simulink model "Aero_Var120"  (R2016b)
settings: Solver=VariableStepAuto  StartTime=0.0  StopTime=10.0  RelTol=1e-3
undefined symbols (not defined in the file or in its folder): AC
libraries: OpenFlightUtilLib x3, simulink x1
settings Model: Creator=UAVLAB  LastModifiedBy=rega0051
settings DataIOCC: ExternalInput=simIn  InitialState=simStateInit  SaveOutput=off  SignalLogging=off  DSMLogging=off  SaveTime=off  StateSaveName=simStates  TimeSaveName=simTime  OutputSaveName=simOut  SignalLoggingName=simLog  DSMLoggingName=simData

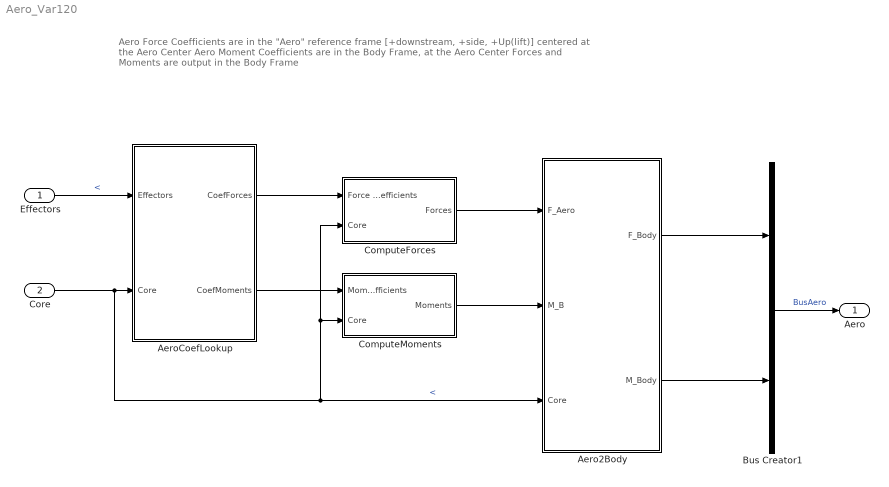
== system Aero_Var120 ==
  note: Aero Force Coefficients are in the "Aero" reference frame [+downstream, +side, +Up(lift)] centered at the Aero Center
      | Aero Moment Coefficients are in the Body Frame, at the Aero Center
      |
      | Forces and Moments are output in the Body Frame
  Effectors : Inport  OutDataTypeStr=Bus: BusEff
      settings: AttributesFormatString=%<OutDataTypeStr>
  Core : Inport  Port=2  OutDataTypeStr=Bus: BusCore
      settings: AttributesFormatString=%<OutDataTypeStr>
  Aero2Body : Subsystem
  AeroCoefLookup : Subsystem
  Bus Creator1 : BusCreator  Inputs=2  OutDataTypeStr=Bus: BusAero
      settings: AttributesFormatString=%<OutDataTypeStr>
  ComputeForces : Subsystem
  ComputeMoments : Subsystem
  Aero : Outport  OutDataTypeStr=Bus: BusAero
      settings: AttributesFormatString=%<OutDataTypeStr>
  wires:
  Effectors/1 -> AeroCoefLookup/1(Effectors)  "<"
  ComputeForces/1(Forces) -> Aero2Body/1(F_Aero)
  ComputeMoments/1(Moments) -> Aero2Body/2(M_B)
  Aero2Body/1(F_Body) -> Bus Creator1/1
  Aero2Body/2(M_Body) -> Bus Creator1/2
  AeroCoefLookup/1(CoefForces) -> ComputeForces/1(Force Coefficients)
  AeroCoefLookup/2(CoefMoments) -> ComputeMoments/1(Moment Coefficients)
  Bus Creator1/1 -> Aero/1  "BusAero"
  Core/1 -> AeroCoefLookup/2(Core), ComputeForces/2(Core), ComputeMoments/2(Core), Aero2Body/3(Core)  "<"

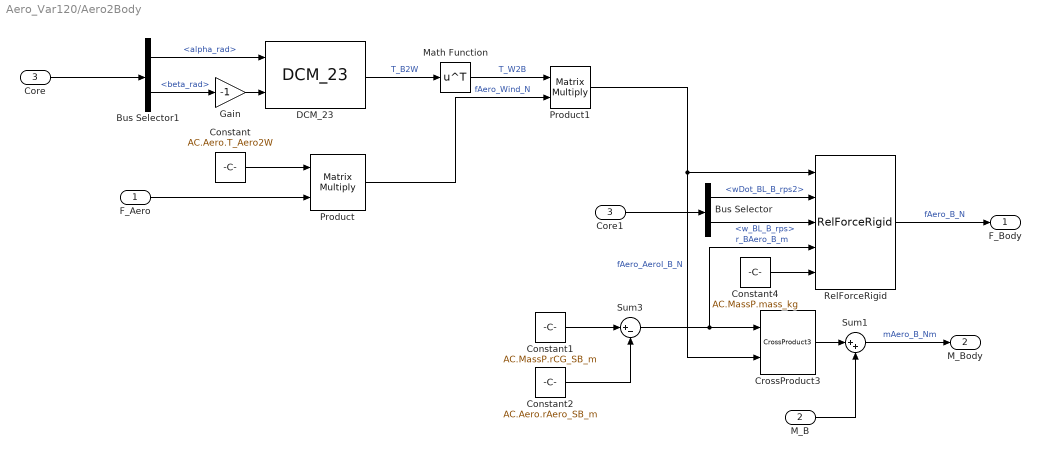
== system Aero_Var120/Aero2Body ==
  F_Aero : Inport
  M_B : Inport  Port=2
  Core : Inport  Port=3
  Bus Selector : BusSelector  OutputSignals=BusEom.wDot_BL_B_rps2,BusEom.w_BL_B_rps
  Bus Selector1 : BusSelector  OutputSignals=BusAux.BusFlow.alpha_rad,BusAux.BusFlow.beta_rad
  Constant : Constant  Value=AC.Aero.T_Aero2W
      settings: AttributesFormatString=%<Value>
  Constant1 : Constant  Value=AC.MassP.rCG_SB_m
      settings: AttributesFormatString=%<Value>
  Constant2 : Constant  Value=AC.Aero.rAero_SB_m
      settings: AttributesFormatString=%<Value>
  Constant4 : Constant  Value=AC.MassP.mass_kg
      settings: AttributesFormatString=%<Value>
  Core1 : InportShadow  Port=3
  CrossProduct3 : OpenFlightUtilLib/Math/CrossProduct3
  DCM_23 : OpenFlightUtilLib/Transformations/DCM_23
  Gain : Gain  Gain=-1
  Math Function : Math  Operator=transpose  SaturateOnIntegerOverflow=on
  Product : Product  Multiplication=Matrix(*)  RndMeth=Zero
  Product1 : Product  Multiplication=Matrix(*)  RndMeth=Zero
  RelForceRigid : OpenFlightUtilLib/Kinematics and Dynamics/RelForceRigid
  Sum1 : Sum  Inputs=|++  SaturateOnIntegerOverflow=on
  Sum3 : Sum  Inputs=|+-  SaturateOnIntegerOverflow=on
  F_Body : Outport
  M_Body : Outport  Port=2
  wires:
  Constant1/1 -> Sum3/1
  Constant2/1 -> Sum3/2
  Bus Selector/1 -> RelForceRigid/2  "<wDot_BL_B_rps2>"
  Bus Selector/2 -> RelForceRigid/3  "<w_BL_B_rps>"
  F_Aero/1 -> Product/2
  Constant/1 -> Product/1
  Core/1 -> Bus Selector1/1
  Math Function/1 -> Product1/1  "T_W2B"
  DCM_23/1 -> Math Function/1  "T_B2W"
  Product/1 -> Product1/2  "fAero_Wind_N"
  Product1/1 -> CrossProduct3/2, RelForceRigid/1  "fAero_AeroI_B_N"
  Sum3/1 -> RelForceRigid/4, CrossProduct3/1  "r_BAero_B_m"
  Core1/1 -> Bus Selector/1
  RelForceRigid/1 -> F_Body/1  "fAero_B_N"
  M_B/1 -> Sum1/2
  CrossProduct3/1 -> Sum1/1
  Sum1/1 -> M_Body/1  "mAero_B_Nm"
  Constant4/1 -> RelForceRigid/5
  Bus Selector1/1 -> DCM_23/1  "<alpha_rad>"
  Bus Selector1/2 -> Gain/1  "<beta_rad>"
  Gain/1 -> DCM_23/2

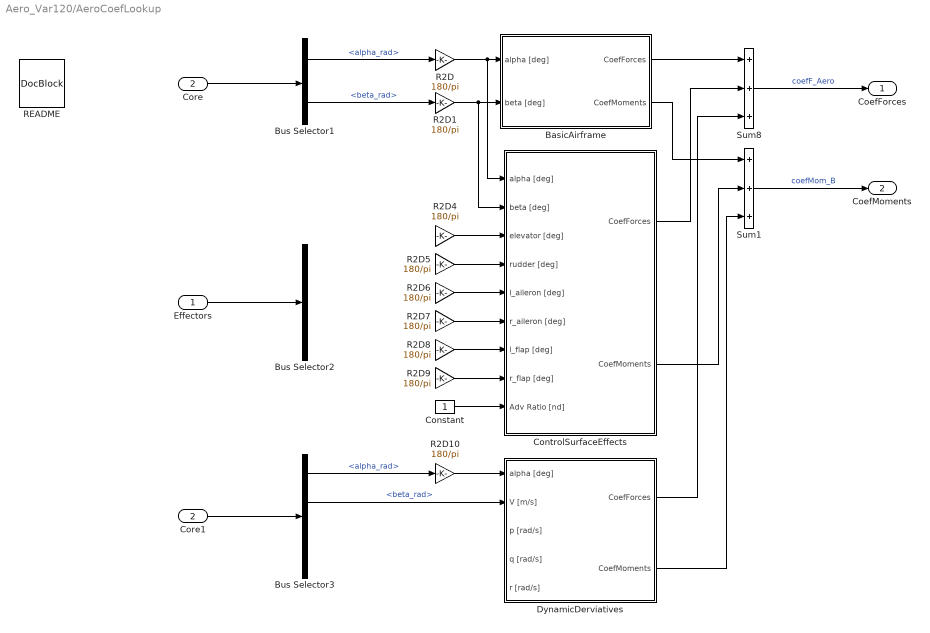
== system Aero_Var120/AeroCoefLookup ==
  Effectors : Inport
  Core : Inport  Port=2
  BasicAirframe : Subsystem
  Bus Selector1 : BusSelector  OutputSignals=BusAux.BusFlow.alpha_rad,BusAux.BusFlow.beta_rad
  Bus Selector2 : BusSelector  OutputSignals=BusSurf
  Bus Selector3 : BusSelector  OutputSignals=BusAux.BusFlow.alpha_rad,BusAux.BusFlow.beta_rad,BusAux.BusFlow.alphaDot_rps,BusAux.BusFlow.betaDot_rps
  Constant : Constant
  ControlSurfaceEffects : Subsystem
  Core1 : InportShadow  Port=2
  DynamicDerviatives : Subsystem
  R2D{,1,4..10} (9 alike) : Gain  Gain=180/pi
  README : simulink/Model-Wide Utilities/DocBlock  DocumentType=Text
      content=|
      | FASER Aerodynamic Model
      |
      | This block models the FASER aerodynamics using a nonlinear, lookup table
      | based, incremental aerodynamic model. This model is based on wind tunnel
      | data obtained from NASA Langley Research Center's 12-Foot Low Speed
      | Tunnel in 2006 and 2011. In general, the baseline aerodynamics are
      | modeled as a nonlinear function of angle of attack and sideslip angle.
      | Control surface effects are modeled as nonlinear functions of angle of
      | attack, sideslip angle, control surface deflection, and advance ratio.
      | Thrust effects are also modeled. DATCOM estimates of linear dynamic
      | derivatives are used for the pitch damping (Cmq), while the effect of
      | roll and yaw rate on CY, Cl, and Cn are modeled as nonlinear functions of
      | angle of attack and nondimensional rate based on forced oscilation wind
      | tunnel data.
      |
      | The effects of control surfaces and rates are modeled for only those
      | coefficients where there was a significant effect observed in the wind
      | tunnel data. They are listed here:
      |
      | Elevator: CD,CL,Cm
      | Rudder: CY,Cn
      | Aileron: Cl
      | Flaps: CD,CL,Cm
      | Thrust: All
      | Roll Rate (p): CY,Cl,Cn
      | Pitch Rate (q): Cm
      | Yaw Rate (r): CY,Cl,Cn
      |
      | The aero tables are stored in \Libraries\FASER_Aero.mat, and are loaded
      | into the aircraft configuration data structure (AC) when the FASER option
      | is input to UAV_config.m.
      |
      | >> AC.Aero
      |
      | ans =
      |
      |            dampder: [1x1 struct]
      |             C6_bas: [1x1 struct]
      |            dC1_ail: [1x1 struct]
      |            dC6_pow: [1x1 struct]
      |           dC3_flap: [1x1 struct]
      |            dC2_rud: [1x1 struct]
      |            dC3_ele: [1x1 struct]
      |              dC3_p: [1x1 struct]
      |              dC3_r: [1x1 struct]
      |     use_FASER_aero: 1
      |
      | The aero data is in the stability axis, so the six aero coefficients are
      | CL, CD, CY, Cl, Cm, Cn. The aero model uses a incremental approach; the
      | basic airframe is modeled in C6_bas; incremental (deltas) effects of
      | control surfaces, angular rate (dampder), and thrust are then added. The
      | form of the data structures is generally as follows:
      |
      | >> AC.Aero.C6_bas
      |
      | ans =
      |
      |      data: [16x13x6 double]
      |     alpha: [-5 0 5 10 11.7500 12.5000 13.2500 13.5000 15 16 17.5000 20 25 30 35 40]
      |      beta: [-30 -25 -20 -15 -10 -5 0 5 10 15 20 25 30]
      |       dim: 'Dimensions are [alpha]x[beta]x[CD,CY,CL,Cl,Cm,Cn]'
      |
      | Currently, the thrust effects are disabled (by setting the advance ratio
      | input to 1), as the current motor model does not output advance ratio.
      |
      | Note on table implementation: pre-lookups on the table indices (eg alpha,
      | beta, etc) are done to increase the speed of the simulation.
  Sum1 : Sum  Inputs=+++  SaturateOnIntegerOverflow=on  InputSameDT=on  OutDataTypeStr=Inherit: Same as first input
  Sum8 : Sum  Inputs=+++  SaturateOnIntegerOverflow=on  InputSameDT=on  OutDataTypeStr=Inherit: Same as first input
  CoefForces : Outport
  CoefMoments : Outport  Port=2
  wires:
  Sum1/1 -> CoefMoments/1  "coefMom_B"
  Sum8/1 -> CoefForces/1  "coefF_Aero"
  Effectors/1 -> Bus Selector2/1
  R2D10/1 -> DynamicDerviatives/1(alpha [deg])
  ? -> DynamicDerviatives/5(r [rad/s])
  ? -> DynamicDerviatives/4(q [rad/s])
  ? -> DynamicDerviatives/3(p [rad/s])
  ? -> R2D4/1
  Constant/1 -> ControlSurfaceEffects/9(Adv Ratio [nd])
  R2D/1 -> ControlSurfaceEffects/1(alpha [deg]), BasicAirframe/1(alpha [deg])
  R2D1/1 -> ControlSurfaceEffects/2(beta [deg]), BasicAirframe/2(beta [deg])
  R2D4/1 -> ControlSurfaceEffects/3(elevator [deg])
  ? -> R2D5/1
  R2D5/1 -> ControlSurfaceEffects/4(rudder [deg])
  ? -> R2D6/1
  ? -> R2D7/1
  ? -> R2D8/1
  ? -> R2D9/1
  R2D6/1 -> ControlSurfaceEffects/5(l_aileron [deg])
  R2D7/1 -> ControlSurfaceEffects/6(r_aileron [deg])
  R2D8/1 -> ControlSurfaceEffects/7(l_flap [deg])
  R2D9/1 -> ControlSurfaceEffects/8(r_flap [deg])
  Bus Selector1/2 -> R2D1/1  "<beta_rad>"
  Bus Selector1/1 -> R2D/1  "<alpha_rad>"
  Bus Selector3/1 -> R2D10/1  "<alpha_rad>"
  Bus Selector3/2 -> DynamicDerviatives/2(V [m/s])  "<beta_rad>"
  Core/1 -> Bus Selector1/1
  Core1/1 -> Bus Selector3/1
  BasicAirframe/1(CoefForces) -> Sum8/1
  ControlSurfaceEffects/1(CoefForces) -> Sum8/2
  DynamicDerviatives/1(CoefForces) -> Sum8/3
  BasicAirframe/2(CoefMoments) -> Sum1/1
  ControlSurfaceEffects/2(CoefMoments) -> Sum1/2
  DynamicDerviatives/2(CoefMoments) -> Sum1/3

== system Aero_Var120/ComputeForces ==
  Force Coefficients : Inport
  Core : Inport  Port=2
  Bus Selector : BusSelector  OutputSignals=BusAux.BusFlow.qBar_Pa
  Demux3 : Demux  Outputs=3
  Gain2 : Gain  Gain=AC.Aero.S  SaturateOnIntegerOverflow=on  OutDataTypeStr=Inherit: Same as input  ParamDataTypeStr=Inherit: Same as input
      settings: AttributesFormatString=%<Gain>
  Mux1 : Mux  Inputs=3
  Product6 : Product  SaturateOnIntegerOverflow=on  InputSameDT=on  OutDataTypeStr=Inherit: Same as first input
  Product7 : Product  SaturateOnIntegerOverflow=on  InputSameDT=on  OutDataTypeStr=Inherit: Same as first input
  Product8 : Product  SaturateOnIntegerOverflow=on  InputSameDT=on  OutDataTypeStr=Inherit: Same as first input
  Forces : Outport
  wires:
  Product6/1 -> Mux1/1  "fD_N"
  Product8/1 -> Mux1/3  "fL_N"
  Product7/1 -> Mux1/2  "fY_N"
  Mux1/1 -> Forces/1  "fAero_N"
  Demux3/2 -> Product7/1  "cY"
  Demux3/1 -> Product6/1  "cD"
  Demux3/3 -> Product8/1  "cL"
  Force Coefficients/1 -> Demux3/1
  Gain2/1 -> Product6/2, Product7/2, Product8/2
  Bus Selector/1 -> Gain2/1  "<qBar_Pa>"
  Core/1 -> Bus Selector/1

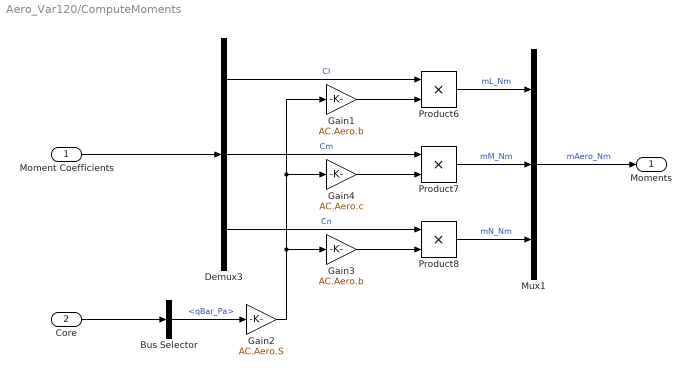
== system Aero_Var120/ComputeMoments ==
  Moment Coefficients : Inport
  Core : Inport  Port=2
  Bus Selector : BusSelector  OutputSignals=BusAux.BusFlow.qBar_Pa
  Demux3 : Demux  Outputs=3
  Gain1 : Gain  Gain=AC.Aero.b  SaturateOnIntegerOverflow=on  OutDataTypeStr=Inherit: Same as input  ParamDataTypeStr=Inherit: Same as input
      settings: AttributesFormatString=%<Gain>
  Gain2 : Gain  Gain=AC.Aero.S  SaturateOnIntegerOverflow=on  OutDataTypeStr=Inherit: Same as input  ParamDataTypeStr=Inherit: Same as input
      settings: AttributesFormatString=%<Gain>
  Gain3 : Gain  Gain=AC.Aero.b  SaturateOnIntegerOverflow=on  OutDataTypeStr=Inherit: Same as input  ParamDataTypeStr=Inherit: Same as input
      settings: AttributesFormatString=%<Gain>
  Gain4 : Gain  Gain=AC.Aero.c  SaturateOnIntegerOverflow=on  OutDataTypeStr=Inherit: Same as input  ParamDataTypeStr=Inherit: Same as input
      settings: AttributesFormatString=%<Gain>
  Mux1 : Mux  Inputs=3
  Product6 : Product  SaturateOnIntegerOverflow=on  InputSameDT=on  OutDataTypeStr=Inherit: Same as first input
  Product7 : Product  SaturateOnIntegerOverflow=on  InputSameDT=on  OutDataTypeStr=Inherit: Same as first input
  Product8 : Product  SaturateOnIntegerOverflow=on  InputSameDT=on  OutDataTypeStr=Inherit: Same as first input
  Moments : Outport
  wires:
  Product6/1 -> Mux1/1  "mL_Nm"
  Product8/1 -> Mux1/3  "mN_Nm"
  Moment Coefficients/1 -> Demux3/1
  Product7/1 -> Mux1/2  "mM_Nm"
  Gain3/1 -> Product8/2
  Mux1/1 -> Moments/1  "mAero_Nm"
  Gain1/1 -> Product6/2
  Gain2/1 -> Gain1/1, Gain4/1, Gain3/1
  Demux3/2 -> Product7/1  "Cm"
  Gain4/1 -> Product7/2
  Demux3/1 -> Product6/1  "Cl"
  Demux3/3 -> Product8/1  "Cn"
  Bus Selector/1 -> Gain2/1  "<qBar_Pa>"
  Core/1 -> Bus Selector/1

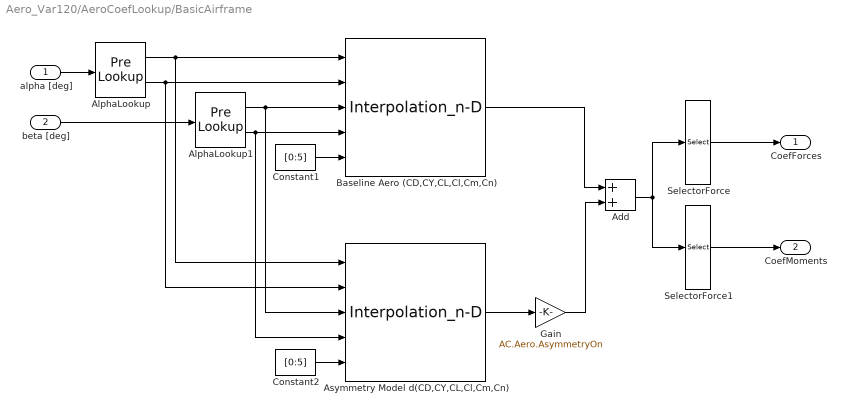
== system Aero_Var120/AeroCoefLookup/BasicAirframe ==
  alpha [deg] : Inport
  beta [deg] : Inport  Port=2
  Add : Sum
  AlphaLookup : PreLookup  BreakpointsData=AC.Aero.C6_bas.alpha  IndexSearchMethod=Linear search  BeginIndexSearchUsingPreviousIndexResult=on  ExtrapMethod=Linear
  AlphaLookup1 : PreLookup  BreakpointsData=AC.Aero.C6_bas.beta  IndexSearchMethod=Linear search  BeginIndexSearchUsingPreviousIndexResult=on  ExtrapMethod=Linear
  Asymmetry Model d(CD,CY,CL,Cl,Cm,Cn) : Interpolation_n-D  NumberOfTableDimensions=3  Table=AC.Aero.dC6_asym.data  NumSelectionDims=1
      settings: InputPortMap=u0,u1,u2,u3,u4
  Baseline Aero (CD,CY,CL,Cl,Cm,Cn) : Interpolation_n-D  NumberOfTableDimensions=3  Table=AC.Aero.C6_bas.data  NumSelectionDims=1
      settings: InputPortMap=u0,u1,u2,u3,u4
  Constant1 : Constant  Value=[0:5]  OutDataTypeStr=uint32
  Constant2 : Constant  Value=[0:5]  OutDataTypeStr=uint32
  Gain : Gain  Gain=AC.Aero.AsymmetryOn
  SelectorForce : Selector  InputPortWidth=6  IndexOptions=Index vector (dialog)  Indices=1:3  OutputSizes=1
  SelectorForce1 : Selector  InputPortWidth=6  IndexOptions=Index vector (dialog)  Indices=1:3  OutputSizes=1
  CoefForces : Outport
  CoefMoments : Outport  Port=2
  wires:
  Constant2/1 -> Asymmetry Model d(CD,CY,CL,Cl,Cm,Cn)/5
  Constant1/1 -> Baseline Aero (CD,CY,CL,Cl,Cm,Cn)/5
  AlphaLookup1/2 -> Asymmetry Model d(CD,CY,CL,Cl,Cm,Cn)/4, Baseline Aero (CD,CY,CL,Cl,Cm,Cn)/4
  AlphaLookup1/1 -> Asymmetry Model d(CD,CY,CL,Cl,Cm,Cn)/3, Baseline Aero (CD,CY,CL,Cl,Cm,Cn)/3
  AlphaLookup/2 -> Asymmetry Model d(CD,CY,CL,Cl,Cm,Cn)/2, Baseline Aero (CD,CY,CL,Cl,Cm,Cn)/2
  AlphaLookup/1 -> Asymmetry Model d(CD,CY,CL,Cl,Cm,Cn)/1, Baseline Aero (CD,CY,CL,Cl,Cm,Cn)/1
  beta [deg]/1 -> AlphaLookup1/1
  alpha [deg]/1 -> AlphaLookup/1
  Asymmetry Model d(CD,CY,CL,Cl,Cm,Cn)/1 -> Gain/1
  Baseline Aero (CD,CY,CL,Cl,Cm,Cn)/1 -> Add/1
  Gain/1 -> Add/2
  Add/1 -> SelectorForce/1, SelectorForce1/1
  SelectorForce/1 -> CoefForces/1
  SelectorForce1/1 -> CoefMoments/1

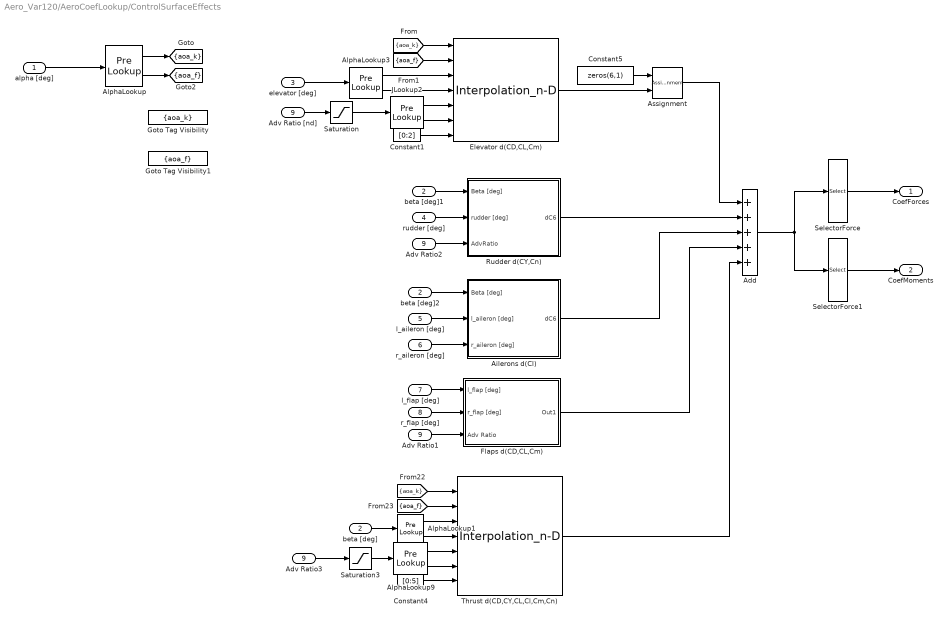
== system Aero_Var120/AeroCoefLookup/ControlSurfaceEffects ==
  alpha [deg] : Inport
  beta [deg] : Inport  Port=2  PortDimensions=1
  elevator [deg] : Inport  Port=3  PortDimensions=1
  rudder [deg] : Inport  Port=4  PortDimensions=1
  l_aileron [deg] : Inport  Port=5  PortDimensions=1
  r_aileron [deg] : Inport  Port=6  PortDimensions=1
  l_flap [deg] : Inport  Port=7  PortDimensions=1
  r_flap [deg] : Inport  Port=8  PortDimensions=1
  Adv Ratio [nd] : Inport  Port=9
  Add : Sum  Inputs=+++++
  Adv Ratio1 : InportShadow  Port=9
  Adv Ratio2 : InportShadow  Port=9
  Adv Ratio3 : InportShadow  Port=9
  Ailerons d(Cl) : Subsystem
  AlphaLookup : PreLookup  BreakpointsData=AC.Aero.C6_bas.alpha  IndexSearchMethod=Linear search  BeginIndexSearchUsingPreviousIndexResult=on  ExtrapMethod=Linear  UseLastBreakpoint=on
  AlphaLookup1 : PreLookup  BreakpointsData=AC.Aero.C6_bas.beta  IndexSearchMethod=Linear search  BeginIndexSearchUsingPreviousIndexResult=on  ExtrapMethod=Linear  UseLastBreakpoint=on
  AlphaLookup3 : PreLookup  BreakpointsData=AC.Aero.dC3_ele.ele  IndexSearchMethod=Linear search  BeginIndexSearchUsingPreviousIndexResult=on  ExtrapMethod=Linear  UseLastBreakpoint=on
  AlphaLookup9 : PreLookup  BreakpointsData=AC.Aero.dC6_pow.J  IndexSearchMethod=Linear search  BeginIndexSearchUsingPreviousIndexResult=on  ExtrapMethod=Linear  UseLastBreakpoint=on
  Assignment : Assignment  IndexOptions=Index vector (dialog)  Indices=[1 3 5]  OutputSizes=[1 1]
  Constant1 : Constant  Value=[0:2]  OutDataTypeStr=uint32
  Constant4 : Constant  Value=[0:5]  OutDataTypeStr=uint32
  Constant5 : Constant  Value=zeros(6,1)
  Elevator d(CD,CL,Cm) : Interpolation_n-D  NumberOfTableDimensions=4  Table=AC.Aero.dC3_ele.data  NumSelectionDims=1
      settings: InputPortMap=u0,u1,u2,u3,u4,u5,u6
  Flaps d(CD,CL,Cm) : Subsystem
  Goto Tag Visibility : GotoTagVisibility  GotoTag=aoa_k
  Goto Tag Visibility1 : GotoTagVisibility  GotoTag=aoa_f
  JLookup2 : PreLookup  BreakpointsData=AC.Aero.dC3_ele.J  IndexSearchMethod=Linear search  BeginIndexSearchUsingPreviousIndexResult=on  ExtrapMethod=Linear  UseLastBreakpoint=on
  Rudder d(CY,Cn) : Subsystem
  Saturation : Saturate  UpperLimit=max(AC.Aero.dC3_ele.J)  LowerLimit=min(AC.Aero.dC3_ele.J)
  Saturation3 : Saturate  UpperLimit=max(AC.Aero.dC6_pow.J)+eps  LowerLimit=min(AC.Aero.dC6_pow.J)+eps
  SelectorForce : Selector  InputPortWidth=6  IndexOptions=Index vector (dialog)  Indices=1:3  OutputSizes=1
  SelectorForce1 : Selector  InputPortWidth=6  IndexOptions=Index vector (dialog)  Indices=1:3  OutputSizes=1
  Thrust d(CD,CY,CL,Cl,Cm,Cn) : Interpolation_n-D  NumberOfTableDimensions=4  Table=AC.Aero.dC6_pow.data  NumSelectionDims=1
      settings: InputPortMap=u0,u1,u2,u3,u4,u5,u6
  beta [deg]1 : InportShadow  Port=2  PortDimensions=1
  beta [deg]2 : InportShadow  Port=2  PortDimensions=1
  CoefForces : Outport
  CoefMoments : Outport  Port=2
  tag scope: aoa_f=scoped, aoa_k=scoped
  wires:
  Thrust d(CD,CY,CL,Cl,Cm,Cn)/1 -> Add/5
  Flaps d(CD,CL,Cm)/1(Out1) -> Add/4
  Ailerons d(Cl)/1(dC6) -> Add/3
  Rudder d(CY,Cn)/1(dC6) -> Add/2
  l_flap [deg]/1 -> Flaps d(CD,CL,Cm)/1(l_flap [deg])
  r_flap [deg]/1 -> Flaps d(CD,CL,Cm)/2(r_flap [deg])
  Adv Ratio1/1 -> Flaps d(CD,CL,Cm)/3(Adv Ratio)
  beta [deg]2/1 -> Ailerons d(Cl)/1(Beta [deg])
  l_aileron [deg]/1 -> Ailerons d(Cl)/2(l_aileron [deg])
  r_aileron [deg]/1 -> Ailerons d(Cl)/3(r_aileron [deg])
  Adv Ratio2/1 -> Rudder d(CY,Cn)/3(AdvRatio)
  rudder [deg]/1 -> Rudder d(CY,Cn)/2(rudder [deg])
  beta [deg]1/1 -> Rudder d(CY,Cn)/1(Beta [deg])
  Saturation3/1 -> AlphaLookup9/1
  Saturation/1 -> JLookup2/1
  Adv Ratio [nd]/1 -> Saturation/1
  Adv Ratio3/1 -> Saturation3/1
  AlphaLookup9/2 -> Thrust d(CD,CY,CL,Cl,Cm,Cn)/6
  AlphaLookup9/1 -> Thrust d(CD,CY,CL,Cl,Cm,Cn)/5
  JLookup2/2 -> Elevator d(CD,CL,Cm)/6
  JLookup2/1 -> Elevator d(CD,CL,Cm)/5
  Assignment/1 -> Add/1
  Constant5/1 -> Assignment/1
  Elevator d(CD,CL,Cm)/1 -> Assignment/2
  Constant4/1 -> Thrust d(CD,CY,CL,Cl,Cm,Cn)/7
  AlphaLookup1/2 -> Thrust d(CD,CY,CL,Cl,Cm,Cn)/4
  AlphaLookup1/1 -> Thrust d(CD,CY,CL,Cl,Cm,Cn)/3
  [aoa_f] -> Thrust d(CD,CY,CL,Cl,Cm,Cn)/2
  [aoa_k] -> Thrust d(CD,CY,CL,Cl,Cm,Cn)/1
  AlphaLookup3/2 -> Elevator d(CD,CL,Cm)/4
  AlphaLookup3/1 -> Elevator d(CD,CL,Cm)/3
  elevator [deg]/1 -> AlphaLookup3/1
  [aoa_f] -> Elevator d(CD,CL,Cm)/2
  [aoa_k] -> Elevator d(CD,CL,Cm)/1
  Constant1/1 -> Elevator d(CD,CL,Cm)/7
  AlphaLookup/2 -> [aoa_f]
  AlphaLookup/1 -> [aoa_k]
  beta [deg]/1 -> AlphaLookup1/1
  alpha [deg]/1 -> AlphaLookup/1
  SelectorForce/1 -> CoefForces/1
  SelectorForce1/1 -> CoefMoments/1
  Add/1 -> SelectorForce/1, SelectorForce1/1

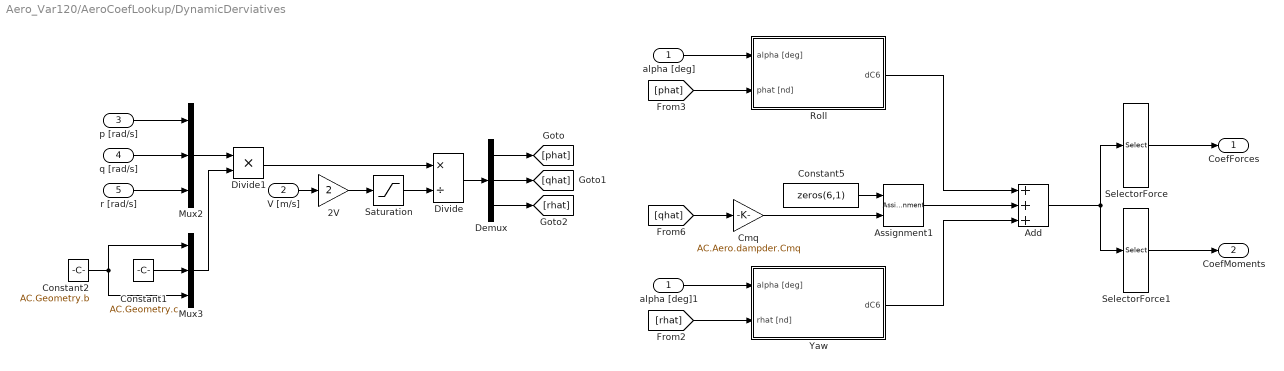
== system Aero_Var120/AeroCoefLookup/DynamicDerviatives ==
  alpha [deg] : Inport
  V [m/s] : Inport  Port=2
  p [rad/s] : Inport  Port=3
  q [rad/s] : Inport  Port=4
  r [rad/s] : Inport  Port=5
  2V : Gain  Gain=2
  Add : Sum  Inputs=+++
  Assignment1 : Assignment  IndexOptions=Index vector (dialog)  Indices=5  OutputSizes=[1 1]
  Cmq : Gain  Gain=AC.Aero.dampder.Cmq
  Constant1 : Constant  Value=AC.Geometry.c
  Constant2 : Constant  Value=AC.Geometry.b
  Constant5 : Constant  Value=zeros(6,1)
  Demux : Demux  Outputs=3
  Divide : Product  Inputs=*/
  Divide1 : Product  Inputs=**
  Mux2 : Mux  Inputs=3
  Mux3 : Mux  Inputs=3
  Roll : Subsystem
  Saturation : Saturate  UpperLimit=Inf  LowerLimit=0.001
  SelectorForce : Selector  InputPortWidth=6  IndexOptions=Index vector (dialog)  Indices=1:3  OutputSizes=1
  SelectorForce1 : Selector  InputPortWidth=6  IndexOptions=Index vector (dialog)  Indices=1:3  OutputSizes=1
  Yaw : Subsystem
  alpha [deg]1 : InportShadow
  CoefForces : Outport
  CoefMoments : Outport  Port=2
  wires:
  Constant2/1 -> Mux3/3, Mux3/1
  Constant1/1 -> Mux3/2
  r [rad/s]/1 -> Mux2/3
  q [rad/s]/1 -> Mux2/2
  p [rad/s]/1 -> Mux2/1
  Mux3/1 -> Divide1/2
  Divide1/1 -> Divide/1
  Mux2/1 -> Divide1/1
  Demux/3 -> [rhat]
  Demux/2 -> [qhat]
  Demux/1 -> [phat]
  Divide/1 -> Demux/1
  Saturation/1 -> Divide/2
  2V/1 -> Saturation/1
  V [m/s]/1 -> 2V/1
  Add/1 -> SelectorForce1/1, SelectorForce/1
  [qhat] -> Cmq/1
  Cmq/1 -> Assignment1/2
  [phat] -> Roll/2(phat [nd])
  [rhat] -> Yaw/2(rhat [nd])
  Constant5/1 -> Assignment1/1
  alpha [deg]/1 -> Roll/1(alpha [deg])
  alpha [deg]1/1 -> Yaw/1(alpha [deg])
  Roll/1(dC6) -> Add/1
  Assignment1/1 -> Add/2
  Yaw/1(dC6) -> Add/3
  SelectorForce/1 -> CoefForces/1
  SelectorForce1/1 -> CoefMoments/1

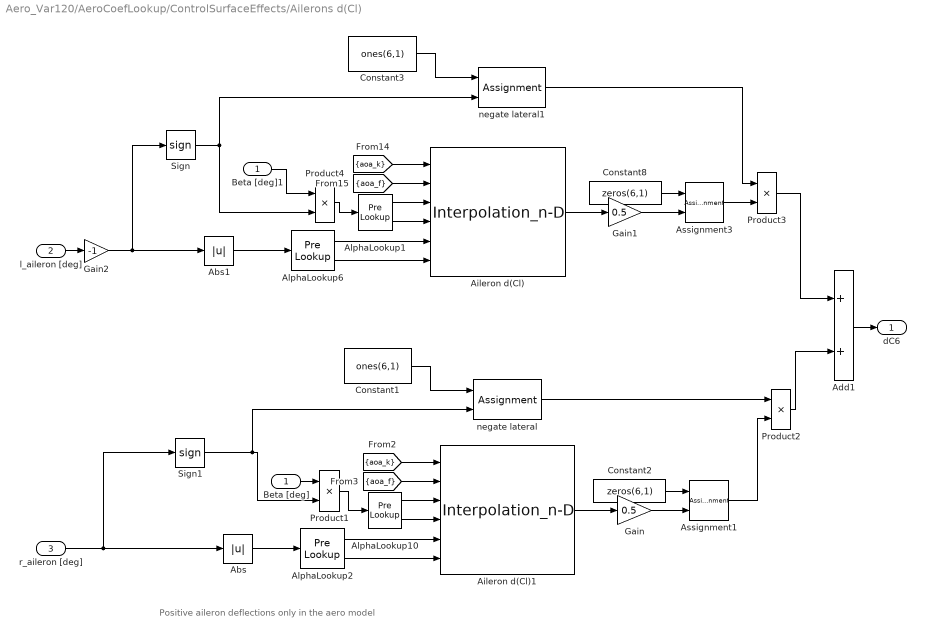
== system Aero_Var120/AeroCoefLookup/ControlSurfaceEffects/Ailerons d(Cl) ==
  note: Positive aileron deflections only in the aero model
  Beta [deg] : Inport  PortDimensions=1
  l_aileron [deg] : Inport  Port=2  PortDimensions=1
  r_aileron [deg] : Inport  Port=3  PortDimensions=1
  Abs : Abs
  Abs1 : Abs
  Add1 : Sum
  Aileron d(Cl) : Interpolation_n-D  NumberOfTableDimensions=3  Table=AC.Aero.dC1_ail.data
      settings: InputPortMap=u0,u1,u2,u3,u4,u5
  Aileron d(Cl)1 : Interpolation_n-D  NumberOfTableDimensions=3  Table=AC.Aero.dC1_ail.data
      settings: InputPortMap=u0,u1,u2,u3,u4,u5
  AlphaLookup1 : PreLookup  BreakpointsData=AC.Aero.dC1_ail.beta  IndexSearchMethod=Linear search  BeginIndexSearchUsingPreviousIndexResult=on  ExtrapMethod=Linear  UseLastBreakpoint=on
  AlphaLookup10 : PreLookup  BreakpointsData=AC.Aero.dC1_ail.beta  IndexSearchMethod=Linear search  BeginIndexSearchUsingPreviousIndexResult=on  ExtrapMethod=Linear  UseLastBreakpoint=on
  AlphaLookup2 : PreLookup  BreakpointsData=AC.Aero.dC1_ail.ail  IndexSearchMethod=Linear search  BeginIndexSearchUsingPreviousIndexResult=on  ExtrapMethod=Linear
  AlphaLookup6 : PreLookup  BreakpointsData=AC.Aero.dC1_ail.ail  IndexSearchMethod=Linear search  BeginIndexSearchUsingPreviousIndexResult=on  ExtrapMethod=Linear
  Assignment1 : Assignment  IndexOptions=Index vector (dialog)  Indices=4  OutputSizes=[1 1]
  Assignment3 : Assignment  IndexOptions=Index vector (dialog)  Indices=4  OutputSizes=[1 1]
  Beta [deg]1 : InportShadow  PortDimensions=1
  Constant1 : Constant  Value=ones(6,1)
  Constant2 : Constant  Value=zeros(6,1)
  Constant3 : Constant  Value=ones(6,1)
  Constant8 : Constant  Value=zeros(6,1)
  Gain : Gain  Gain=0.5
  Gain1 : Gain  Gain=0.5
  Gain2 : Gain  Gain=-1
  Product{1..4} (4 alike) : Product  RndMeth=Zero
  Sign : Signum
  Sign1 : Signum
  negate lateral : Assignment  IndexMode=Zero-based  IndexOptions=Index vector (dialog)  Indices=[1 3 5]  OutputSizes=[1 1]
  negate lateral1 : Assignment  IndexMode=Zero-based  IndexOptions=Index vector (dialog)  Indices=[1 3 5]  OutputSizes=[1 1]
  dC6 : Outport
  wires:
  Gain1/1 -> Assignment3/2
  Gain/1 -> Assignment1/2
  Gain2/1 -> Sign/1, Abs1/1
  Beta [deg]1/1 -> Product4/1
  Sign/1 -> negate lateral1/2, Product4/2
  Product4/1 -> AlphaLookup1/1
  AlphaLookup1/1 -> Aileron d(Cl)/3
  Abs1/1 -> AlphaLookup6/1
  negate lateral1/1 -> Product3/1
  Constant3/1 -> negate lateral1/1
  Product3/1 -> Add1/1
  Assignment3/1 -> Product3/2
  Product2/1 -> Add1/2
  negate lateral/1 -> Product2/1
  Assignment1/1 -> Product2/2
  Aileron d(Cl)1/1 -> Gain/1
  Constant2/1 -> Assignment1/1
  Constant1/1 -> negate lateral/1
  Beta [deg]/1 -> Product1/1
  Sign1/1 -> negate lateral/2, Product1/2
  Product1/1 -> AlphaLookup10/1
  AlphaLookup10/2 -> Aileron d(Cl)1/4
  AlphaLookup10/1 -> Aileron d(Cl)1/3
  Abs/1 -> AlphaLookup2/1
  Add1/1 -> dC6/1
  l_aileron [deg]/1 -> Gain2/1
  r_aileron [deg]/1 -> Sign1/1, Abs/1
  AlphaLookup2/2 -> Aileron d(Cl)1/6
  AlphaLookup2/1 -> Aileron d(Cl)1/5
  [aoa_f] -> Aileron d(Cl)1/2
  [aoa_k] -> Aileron d(Cl)1/1
  Constant8/1 -> Assignment3/1
  Aileron d(Cl)/1 -> Gain1/1
  AlphaLookup6/2 -> Aileron d(Cl)/6
  AlphaLookup6/1 -> Aileron d(Cl)/5
  AlphaLookup1/2 -> Aileron d(Cl)/4
  [aoa_f] -> Aileron d(Cl)/2
  [aoa_k] -> Aileron d(Cl)/1

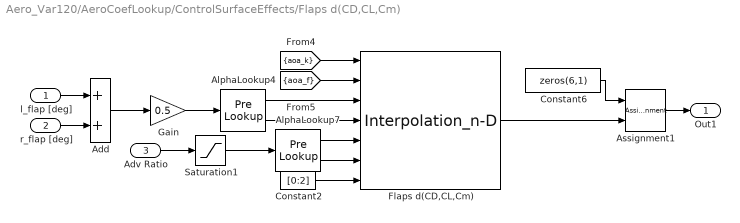
== system Aero_Var120/AeroCoefLookup/ControlSurfaceEffects/Flaps d(CD,CL,Cm) ==
  l_flap [deg] : Inport  PortDimensions=1
  r_flap [deg] : Inport  Port=2  PortDimensions=1
  Adv Ratio : Inport  Port=3
  Add : Sum
  AlphaLookup4 : PreLookup  BreakpointsData=AC.Aero.dC3_flap.flap  IndexSearchMethod=Linear search  BeginIndexSearchUsingPreviousIndexResult=on  ExtrapMethod=Linear
  AlphaLookup7 : PreLookup  BreakpointsData=AC.Aero.dC3_flap.J  IndexSearchMethod=Linear search  BeginIndexSearchUsingPreviousIndexResult=on  ExtrapMethod=Linear  UseLastBreakpoint=on
  Assignment1 : Assignment  IndexOptions=Index vector (dialog)  Indices=[1 3 5]  OutputSizes=[1 1]
  Constant2 : Constant  Value=[0:2]  OutDataTypeStr=uint32
  Constant6 : Constant  Value=zeros(6,1)
  Flaps d(CD,CL,Cm) : Interpolation_n-D  NumberOfTableDimensions=4  Table=AC.Aero.dC3_flap.data  NumSelectionDims=1
      settings: InputPortMap=u0,u1,u2,u3,u4,u5,u6
  Gain : Gain  Gain=0.5
  Saturation1 : Saturate  UpperLimit=max(AC.Aero.dC3_flap.J)  LowerLimit=min(AC.Aero.dC3_flap.J)
  Out1 : Outport
  wires:
  Gain/1 -> AlphaLookup4/1
  Add/1 -> Gain/1
  r_flap [deg]/1 -> Add/2
  l_flap [deg]/1 -> Add/1
  Assignment1/1 -> Out1/1
  Saturation1/1 -> AlphaLookup7/1
  Adv Ratio/1 -> Saturation1/1
  AlphaLookup7/2 -> Flaps d(CD,CL,Cm)/6
  AlphaLookup7/1 -> Flaps d(CD,CL,Cm)/5
  Constant6/1 -> Assignment1/1
  Flaps d(CD,CL,Cm)/1 -> Assignment1/2
  AlphaLookup4/2 -> Flaps d(CD,CL,Cm)/4
  AlphaLookup4/1 -> Flaps d(CD,CL,Cm)/3
  [aoa_f] -> Flaps d(CD,CL,Cm)/2
  [aoa_k] -> Flaps d(CD,CL,Cm)/1
  Constant2/1 -> Flaps d(CD,CL,Cm)/7

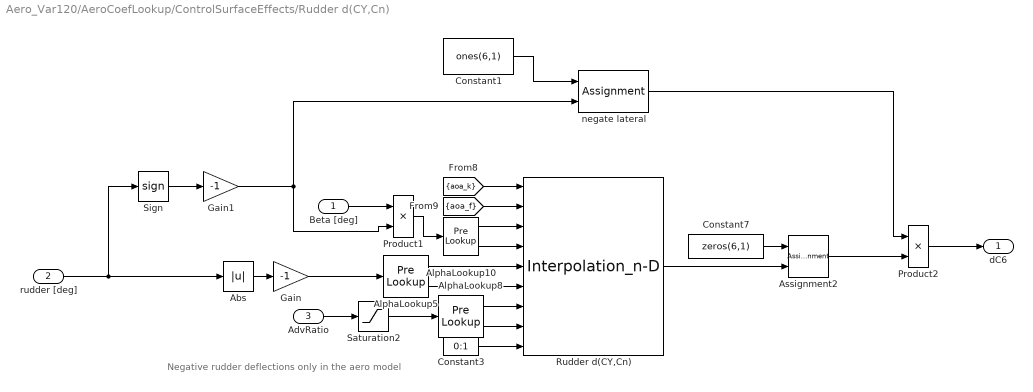
== system Aero_Var120/AeroCoefLookup/ControlSurfaceEffects/Rudder d(CY,Cn) ==
  note: Negative rudder deflections only in the aero model
  Beta [deg] : Inport  PortDimensions=1
  rudder [deg] : Inport  Port=2  PortDimensions=1
  AdvRatio : Inport  Port=3
  Abs : Abs
  AlphaLookup10 : PreLookup  BreakpointsData=AC.Aero.dC2_rud.beta  IndexSearchMethod=Linear search  BeginIndexSearchUsingPreviousIndexResult=on  ExtrapMethod=Linear  UseLastBreakpoint=on
  AlphaLookup5 : PreLookup  BreakpointsData=AC.Aero.dC2_rud.rud  IndexSearchMethod=Linear search  BeginIndexSearchUsingPreviousIndexResult=on  ExtrapMethod=Linear
  AlphaLookup8 : PreLookup  BreakpointsData=AC.Aero.dC2_rud.J  IndexSearchMethod=Linear search  BeginIndexSearchUsingPreviousIndexResult=on  ExtrapMethod=Linear  UseLastBreakpoint=on
  Assignment2 : Assignment  IndexOptions=Index vector (dialog)  Indices=[2 6]  OutputSizes=[1 1]
  Constant1 : Constant  Value=ones(6,1)
  Constant3 : Constant  Value=0:1  OutDataTypeStr=uint32
  Constant7 : Constant  Value=zeros(6,1)
  Gain : Gain  Gain=-1
  Gain1 : Gain  Gain=-1
  Product1 : Product  RndMeth=Zero
  Product2 : Product  RndMeth=Zero
  Rudder d(CY,Cn) : Interpolation_n-D  NumberOfTableDimensions=5  Table=AC.Aero.dC2_rud.data  NumSelectionDims=1
      settings: InputPortMap=u0,u1,u2,u3,u4,u5,u6,u7,u8
  Saturation2 : Saturate  UpperLimit=max(AC.Aero.dC2_rud.J)  LowerLimit=min(AC.Aero.dC2_rud.J)
  Sign : Signum
  negate lateral : Assignment  IndexMode=Zero-based  IndexOptions=Index vector (dialog)  Indices=[1 3 5]  OutputSizes=[1 1]
  dC6 : Outport
  wires:
  Gain1/1 -> negate lateral/2, Product1/2
  negate lateral/1 -> Product2/1
  Assignment2/1 -> Product2/2
  Product2/1 -> dC6/1
  Constant1/1 -> negate lateral/1
  Sign/1 -> Gain1/1
  Product1/1 -> AlphaLookup10/1
  Beta [deg]/1 -> Product1/1
  Gain/1 -> AlphaLookup5/1
  rudder [deg]/1 -> Sign/1, Abs/1
  Abs/1 -> Gain/1
  AlphaLookup10/2 -> Rudder d(CY,Cn)/4
  AlphaLookup10/1 -> Rudder d(CY,Cn)/3
  Saturation2/1 -> AlphaLookup8/1
  AdvRatio/1 -> Saturation2/1
  AlphaLookup8/2 -> Rudder d(CY,Cn)/8
  AlphaLookup8/1 -> Rudder d(CY,Cn)/7
  Constant7/1 -> Assignment2/1
  Rudder d(CY,Cn)/1 -> Assignment2/2
  AlphaLookup5/2 -> Rudder d(CY,Cn)/6
  AlphaLookup5/1 -> Rudder d(CY,Cn)/5
  Constant3/1 -> Rudder d(CY,Cn)/9
  [aoa_f] -> Rudder d(CY,Cn)/2
  [aoa_k] -> Rudder d(CY,Cn)/1

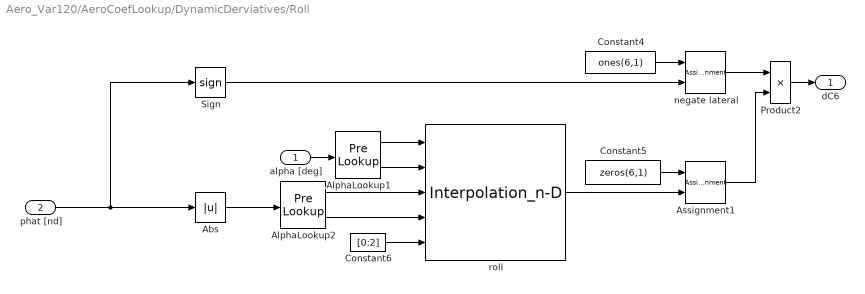
== system Aero_Var120/AeroCoefLookup/DynamicDerviatives/Roll ==
  alpha [deg] : Inport
  phat [nd] : Inport  Port=2
  Abs : Abs
  AlphaLookup1 : PreLookup  BreakpointsData=AC.Aero.dC3_p.alpha  IndexSearchMethod=Linear search  BeginIndexSearchUsingPreviousIndexResult=on  ExtrapMethod=Linear
  AlphaLookup2 : PreLookup  BreakpointsData=AC.Aero.dC3_p.phat  IndexSearchMethod=Linear search  BeginIndexSearchUsingPreviousIndexResult=on  ExtrapMethod=Linear
  Assignment1 : Assignment  IndexOptions=Index vector (dialog)  Indices=[2 4 6]  OutputSizes=[1 1]
  Constant4 : Constant  Value=ones(6,1)
  Constant5 : Constant  Value=zeros(6,1)
  Constant6 : Constant  Value=[0:2]  OutDataTypeStr=uint32
  Product2 : Product  RndMeth=Zero
  Sign : Signum
  negate lateral : Assignment  IndexOptions=Index vector (dialog)  Indices=[2 4 6]  OutputSizes=[1 1]
  roll : Interpolation_n-D  NumberOfTableDimensions=3  Table=AC.Aero.dC3_p.data  NumSelectionDims=1
      settings: InputPortMap=u0,u1,u2,u3,u4
  dC6 : Outport
  wires:
  Sign/1 -> negate lateral/2
  negate lateral/1 -> Product2/1
  Assignment1/1 -> Product2/2
  roll/1 -> Assignment1/2
  Constant5/1 -> Assignment1/1
  Constant4/1 -> negate lateral/1
  Abs/1 -> AlphaLookup2/1
  phat [nd]/1 -> Sign/1, Abs/1
  AlphaLookup2/1 -> roll/3
  AlphaLookup2/2 -> roll/4
  Constant6/1 -> roll/5
  AlphaLookup1/1 -> roll/1
  AlphaLookup1/2 -> roll/2
  Product2/1 -> dC6/1
  alpha [deg]/1 -> AlphaLookup1/1

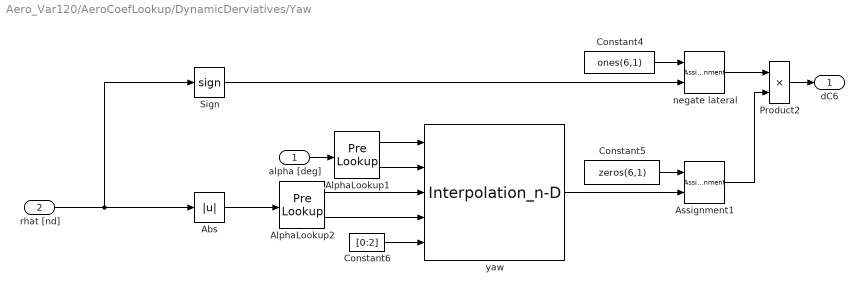
== system Aero_Var120/AeroCoefLookup/DynamicDerviatives/Yaw ==
  alpha [deg] : Inport
  rhat [nd] : Inport  Port=2
  Abs : Abs
  AlphaLookup1 : PreLookup  BreakpointsData=AC.Aero.dC3_r.alpha  IndexSearchMethod=Linear search  BeginIndexSearchUsingPreviousIndexResult=on  ExtrapMethod=Linear
  AlphaLookup2 : PreLookup  BreakpointsData=AC.Aero.dC3_r.rhat  IndexSearchMethod=Linear search  BeginIndexSearchUsingPreviousIndexResult=on  ExtrapMethod=Linear
  Assignment1 : Assignment  IndexOptions=Index vector (dialog)  Indices=[2 4 6]  OutputSizes=[1 1]
  Constant4 : Constant  Value=ones(6,1)
  Constant5 : Constant  Value=zeros(6,1)
  Constant6 : Constant  Value=[0:2]  OutDataTypeStr=uint32
  Product2 : Product  RndMeth=Zero
  Sign : Signum
  negate lateral : Assignment  IndexOptions=Index vector (dialog)  Indices=[2 4 6]  OutputSizes=[1 1]
  yaw : Interpolation_n-D  NumberOfTableDimensions=3  Table=AC.Aero.dC3_r.data  NumSelectionDims=1
      settings: InputPortMap=u0,u1,u2,u3,u4
  dC6 : Outport
  wires:
  Sign/1 -> negate lateral/2
  negate lateral/1 -> Product2/1
  Constant4/1 -> negate lateral/1
  alpha [deg]/1 -> AlphaLookup1/1
  Product2/1 -> dC6/1
  AlphaLookup1/2 -> yaw/2
  AlphaLookup1/1 -> yaw/1
  Constant6/1 -> yaw/5
  AlphaLookup2/2 -> yaw/4
  AlphaLookup2/1 -> yaw/3
  rhat [nd]/1 -> Sign/1, Abs/1
  Abs/1 -> AlphaLookup2/1
  Constant5/1 -> Assignment1/1
  yaw/1 -> Assignment1/2
  Assignment1/1 -> Product2/2
